simulink library "halout"  (R2021b)
settings: Solver=VariableStepAuto  StartTime=0.0  StopTime=10.0  RelTol=1e-3
undefined symbols (not defined in the file): C_TASK_5MS_S, FALSE, KHAL_CAN1TxReq_flg, KHAL_CAN2TxReq_flg, KHAL_CAN3FD3VCU1toNIDECTxReq_flg, KHAL_CAN3FD3VCU1TxReq_flg, KHAL_CAN3FD3VCU2E2E_flg, KHAL_CAN3FD3VCU2toNIDECE2E_flg, KHAL_CAN3FD3VCU2toNIDECTxReq_flg, KHAL_CAN3FD3VCU2TxReq_flg, KHAL_CAN3TxReq_flg, KHAL_CAN4FD4CE1000E2E_flg, KHAL_CAN4FD4CE1000TxReq_flg, KHAL_CAN4TxReq_flg, KHAL_CAN5TxReq_flg, KHAL_CAN7TxReq_flg, ONE_INT, TRUE, ZERO_INT
libraries: FVT_lib x258, simulink x115
(part 7 of 17)

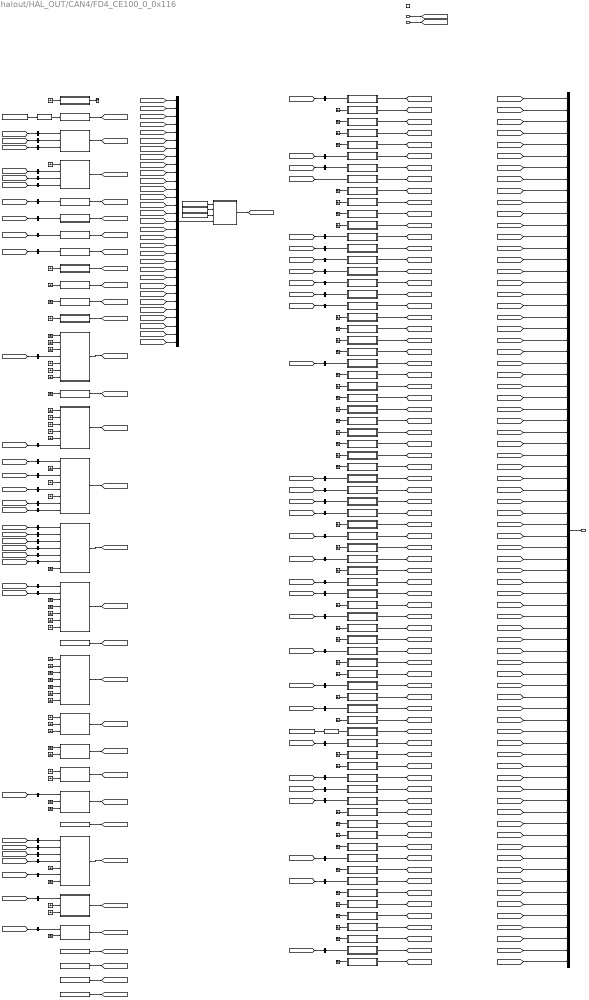
== system halout/HAL_OUT/CAN4/FD4_CE100_0_0x116 ==
  BSCP_outputs : Inport  OutDataTypeStr=Bus: BSCP_outputs
  BOUTP_outputs : Inport  Port=2  OutDataTypeStr=Bus: BOUTP_outputs
  Trigger : TriggerPort  TriggerType=function-call  VariantControl=(inherit)
  APSStaSystem : Subsystem
  AllDoorSW : Subsystem
  AntiTheftSeatFold : Subsystem
  AntitheftSta : Subsystem
  BCMDoorLockSta : Subsystem
  BrakeLamp : Subsystem
  Byte_0 : Subsystem
  Byte_1 : Subsystem
  Byte_10 : Subsystem
  Byte_11 : Subsystem
  Byte_12 : Subsystem
  Byte_13 : Subsystem
  Byte_14 : Subsystem
  Byte_15 : Subsystem
  Byte_16 : Subsystem
  Byte_17 : Subsystem
  Byte_{18,24,28..31} (6 alike) : Constant  Value=ZERO_INT
  Byte_19 : Subsystem
  Byte_2 : Subsystem
  Byte_20 : Subsystem
  Byte_21 : Subsystem
  Byte_22 : Subsystem
  Byte_23 : Subsystem
  Byte_25 : Subsystem
  Byte_26 : Subsystem
  Byte_27 : Subsystem
  Byte_3 : Subsystem
  Byte_4 : Subsystem
  Byte_5 : Subsystem
  Byte_6 : Subsystem
  Byte_7 : Subsystem
  Byte_8 : Subsystem
  Byte_9 : Subsystem
  CCCrlSta : Subsystem
  CRC8_IfAction_Tx : Subsystem  AncestorBlock=FVT_lib/hal/CRC8_IfAction_Tx
      mask help: MeasumentTrigerEvent
      mask Display: fprintf('CRC8_IfAction');
  CSVCU1CAN4 : Subsystem
  CTDCtrl : Subsystem
  CTDLockSW : Subsystem
  CTDUnlockSW : Subsystem
  Constant : Constant  Value=KHAL_CAN4FD4CE1000E2E_flg
  Constant1 : Constant  Value=0x08
  Constant2 : Constant  Value=0x4D
  Constant3 : Constant  Value=KHAL_CAN4FD4CE1000E2E_flg
  Constant4 : Constant  Value=KHAL_CAN4FD4CE1000E2E_flg
  CrashDetd : Subsystem
  CtrlDrPwrStbA2 : Subsystem
  CtrlFrBMSCCUCIR : Subsystem
  CtrlFrEDUINVERTER : Subsystem
  CtrlFrIRC1 : Subsystem
  CtrlFrPwrStbA1P : Subsystem
  DKCAuthSta : Subsystem
  DKCTimeSN : Subsystem
  Dimmer : Subsystem
  DimmerEN : Subsystem
  DoorLockIND : Subsystem
  DrDoorSW : Subsystem
  DrSeatSta : Subsystem
  EquivAccPedalSWSta : Subsystem
  FDDKCVehDataErr : Subsystem
  FDDKCVehDataSta : Subsystem
  FDTBOXDTCDataErr : Subsystem
  FDTBOXDTCDataSta : Subsystem
  FDTBOXVehDataErr : Subsystem
  FDTBOXVehDataSta : Subsystem
  FrChargingDoorCtrl : Subsystem
  FrFogLamp : Subsystem
  FrWiperH : Subsystem
  FrWiperL : Subsystem
  Ground{,1..91} (92 alike) : Ground
  HBeam : Subsystem
  HBeamADB : Subsystem
  HWResetSta : Subsystem
  HazardSW : Subsystem
  HoodSW : Subsystem
  HornCtrl : Subsystem
  LAPMWdwEnable : Subsystem
  LBSD : Subsystem
  LBeam : Subsystem
  LDRL : Subsystem
  LTurnLP : Subsystem
  LampPwr : Subsystem
  LockSetting : Subsystem
  MSACrlSta : Subsystem
  MirrorCtrl : Subsystem
  MirrorDefog : Subsystem
  Mux2 : Mux  Inputs=31
  PosLamp : Subsystem
  PsDoorSW : Subsystem
  PwrSta : Subsystem
  RBSD : Subsystem
  RCVCU1CAN4 : Subsystem
  RDRL : Subsystem
  RLDoorSW : Subsystem
  RRDoorSW : Subsystem
  RTurnLP : Subsystem
  ReBrakeLPReq : Subsystem
  ReverseLamp : Subsystem
  RollingCounter_IfAction : FVT_lib/hal/RollingCounter_IfAction
  RollingCounter_IfAction1 : FVT_lib/hal/RollingCounter_IfAction
  RoomLampH : Subsystem
  RoomLampL : Subsystem
  RrChargingDoorCtrl : Subsystem
  RrDefog : Subsystem
  RrFogLamp : Subsystem
  RrWiper : Subsystem
  ShiftGearPosn : Subsystem
  TailgateHDSW : Subsystem
  TailgateRemote : Subsystem
  TailgateSW : Subsystem
  Terminator : Terminator
  TimeSNDKCFbk : Subsystem
  TrunkRel : Subsystem
  WasherCtrl : Subsystem
  WiperFixMode : Subsystem
  bus_creator : BusCreator  Inputs=76  OutDataTypeStr=Bus: DT_CAN4_SG_FD4_CE100_0  NonVirtualBus=on
  bus_selector : BusSelector  OutputSignals=VOUTP_CCCtrlSta_enum
  bus_selector1 : BusSelector  OutputSignals=VOUTP_DrSeatSta_enum
  bus_selector10 : BusSelector  OutputSignals=VOUTP_HornCtrl_flg
  bus_selector11 : BusSelector  OutputSignals=VOUTP_RTurnLP_flg
  bus_selector12 : BusSelector  OutputSignals=VOUTP_BrakeLamp_flg
  bus_selector13 : BusSelector  OutputSignals=VOUTP_HazardSW_flg
  bus_selector14 : BusSelector  OutputSignals=VOUTP_LTurnLP_flg
  bus_selector15 : BusSelector  OutputSignals=VOUTP_ReverseLamp_flg
  bus_selector16 : BusSelector  OutputSignals=VOUTP_RrFogLamp_flg
  bus_selector17 : BusSelector  OutputSignals=VOUTP_HBeam_flg
  bus_selector18 : BusSelector  OutputSignals=VOUTP_LDRL_flg
  bus_selector19 : BusSelector  OutputSignals=VOUTP_LBeam_flg
  bus_selector2 : BusSelector  OutputSignals=VOUTP_MSACtrlSta_enum
  bus_selector20 : BusSelector  OutputSignals=VOUTP_PosLamp_flg
  bus_selector21 : BusSelector  OutputSignals=VOUTP_RDRL_flg
  bus_selector22 : BusSelector  OutputSignals=VOUTP_WasherCtrl_enum
  bus_selector23 : BusSelector  OutputSignals=VOUTP_FrWiperH_flg
  bus_selector24 : BusSelector  OutputSignals=VOUTP_FrWiperL_flg
  bus_selector25 : BusSelector  OutputSignals=VOUTP_DKCAuthSta_enum
  bus_selector26 : BusSelector  OutputSignals=VOUTP_CtrlFrBMSCCUCIR_flg
  bus_selector27 : BusSelector  OutputSignals=VOUTP_CtrlFrEDUINVERTER_flg
  bus_selector28 : BusSelector  OutputSignals=VOUTP_CtrlFrRC1_flg
  bus_selector29 : BusSelector  OutputSignals=VOUTP_CtrlFrPwrStbA1P_flg
  bus_selector3 : BusSelector  OutputSignals=VOUTP_PowerSta_enum
  bus_selector30 : BusSelector  OutputSignals=VOUTP_HWResetSta_enum
  bus_selector31 : BusSelector  OutputSignals=VOUTP_APSStaSys_enum
  bus_selector32 : BusSelector  OutputSignals=VOUTP_CtrlDrPwrStbA2_flg
  bus_selector33 : BusSelector  OutputSignals=VOUTP_APSStaSys_enum
  bus_selector34 : BusSelector  OutputSignals=VOUTP_BrakeLamp_flg
  bus_selector35 : BusSelector  OutputSignals=VOUTP_CCCtrlSta_enum
  bus_selector36 : BusSelector  OutputSignals=VOUTP_CtrlDrPwrStbA2_flg
  bus_selector37 : BusSelector  OutputSignals=VOUTP_CtrlFrBMSCCUCIR_flg
  bus_selector38 : BusSelector  OutputSignals=VOUTP_CtrlFrEDUINVERTER_flg
  bus_selector39 : BusSelector  OutputSignals=VOUTP_CtrlFrRC1_flg
  bus_selector4 : BusSelector  OutputSignals=VOUTP_ReBrakeLPReq_flg
  bus_selector40 : BusSelector  OutputSignals=VOUTP_CtrlFrPwrStbA1P_flg
  bus_selector41 : BusSelector  OutputSignals=VOUTP_DKCAuthSta_enum
  bus_selector{6..9,42} (5 alike) : BusSelector  OutputSignals=VOUTP_DKCTimeSN_cnt
  bus_selector43 : BusSelector  OutputSignals=VOUTP_DrSeatSta_enum
  bus_selector44 : BusSelector  OutputSignals=VOUTP_FrWiperH_flg
  bus_selector45 : BusSelector  OutputSignals=VOUTP_FrWiperL_flg
  bus_selector46 : BusSelector  OutputSignals=VOUTP_HWResetSta_enum
  bus_selector47 : BusSelector  OutputSignals=VOUTP_HBeam_flg
  bus_selector48 : BusSelector  OutputSignals=VOUTP_HazardSW_flg
  bus_selector49 : BusSelector  OutputSignals=VOUTP_HornCtrl_flg
  bus_selector5 : BusSelector  OutputSignals=VOUTP_ShiftGearPosn_enum
  bus_selector50 : BusSelector  OutputSignals=VOUTP_LDRL_flg
  bus_selector51 : BusSelector  OutputSignals=VOUTP_LTurnLP_flg
  bus_selector52 : BusSelector  OutputSignals=VOUTP_LBeam_flg
  bus_selector53 : BusSelector  OutputSignals=VOUTP_MSACtrlSta_enum
  bus_selector54 : BusSelector  OutputSignals=VOUTP_PosLamp_flg
  bus_selector55 : BusSelector  OutputSignals=VOUTP_PowerSta_enum
  bus_selector56 : BusSelector  OutputSignals=VOUTP_RDRL_flg
  bus_selector57 : BusSelector  OutputSignals=VOUTP_RTurnLP_flg
  bus_selector58 : BusSelector  OutputSignals=VOUTP_ReBrakeLPReq_flg
  bus_selector59 : BusSelector  OutputSignals=VOUTP_ReverseLamp_flg
  bus_selector60 : BusSelector  OutputSignals=VOUTP_RrFogLamp_flg
  bus_selector61 : BusSelector  OutputSignals=VOUTP_ShiftGearPosn_enum
  bus_selector62 : BusSelector  OutputSignals=VOUTP_WasherCtrl_enum
  FD4_CE100_0 : Outport
  wires:
  BSCP_outputs/1 -> [BSCP_outputs]
  BOUTP_outputs/1 -> [BOUTP_outputs]
  [CAN4_APS_Sta_System] -> bus_creator/1  "CAN4_APS_Sta_System"
  [CAN4_AllDoorSW] -> bus_creator/2  "CAN4_AllDoorSW"
  [CAN4_AntiTheftSeatFold] -> bus_creator/3  "CAN4_AntiTheftSeatFold"
  [CAN4_AntitheftSta] -> bus_creator/4  "CAN4_AntitheftSta"
  [CAN4_BCM_DoorLock_Sta] -> bus_creator/5  "CAN4_BCM_DoorLock_Sta"
  [CAN4_BrakeLamp] -> bus_creator/6  "CAN4_BrakeLamp"
  [CAN4_CC_Crl_Sta] -> bus_creator/7  "CAN4_CC_Crl_Sta"
  [CAN4_CS_VCU1_CAN4] -> bus_creator/8  "CAN4_CS_VCU1_CAN4"
  [CAN4_CTDCtrl] -> bus_creator/9  "CAN4_CTDCtrl"
  [CAN4_CTDLockSW] -> bus_creator/10  "CAN4_CTDLockSW"
  [CAN4_CTDUnlockSW] -> bus_creator/11  "CAN4_CTDUnlockSW"
  [CAN4_CrashDetd] -> bus_creator/12  "CAN4_CrashDetd"
  [CAN4_CtrlDrPwrStbA2] -> bus_creator/13  "CAN4_CtrlDrPwrStbA2"
  [CAN4_CtrlFrBMSCCUCIR] -> bus_creator/14  "CAN4_CtrlFrBMSCCUCIR"
  [CAN4_CtrlFrEDUINVERTER] -> bus_creator/15  "CAN4_CtrlFrEDUINVERTER"
  [CAN4_CtrlFrIRC1] -> bus_creator/16  "CAN4_CtrlFrIRC1"
  [CAN4_CtrlFrPwrStbA1P] -> bus_creator/17  "CAN4_CtrlFrPwrStbA1P"
  [CAN4_DKCAuthSta] -> bus_creator/18  "CAN4_DKCAuthSta"
  [CAN4_DKCTimeSN] -> bus_creator/19  "CAN4_DKCTimeSN"
  [CAN4_Dimmer] -> bus_creator/20  "CAN4_Dimmer"
  [CAN4_DimmerEN] -> bus_creator/21  "CAN4_DimmerEN"
  [CAN4_DoorLockIND] -> bus_creator/22  "CAN4_DoorLockIND"
  [CAN4_DrDoorSW] -> bus_creator/23  "CAN4_DrDoorSW"
  [CAN4_Dr_SeatSta] -> bus_creator/24  "CAN4_Dr_SeatSta"
  [CAN4_EquivAccPedalSWSta] -> bus_creator/25  "CAN4_EquivAccPedalSWSta"
  [CAN4_FD_DKC_VehData_Err] -> bus_creator/26  "CAN4_FD_DKC_VehData_Err"
  [CAN4_FD_DKC_VehData_Sta] -> bus_creator/27  "CAN4_FD_DKC_VehData_Sta"
  [CAN4_FD_TBOX_DTCData_Err] -> bus_creator/28  "CAN4_FD_TBOX_DTCData_Err"
  [CAN4_FD_TBOX_DTCData_Sta] -> bus_creator/29  "CAN4_FD_TBOX_DTCData_Sta"
  [CAN4_FD_TBOX_VehData_Err] -> bus_creator/30  "CAN4_FD_TBOX_VehData_Err"
  [CAN4_FD_TBOX_VehData_Sta] -> bus_creator/31  "CAN4_FD_TBOX_VehData_Sta"
  [CAN4_Fr_ChargingDoorCtrl] -> bus_creator/32  "CAN4_Fr_ChargingDoorCtrl"
  [CAN4_Fr_FogLamp] -> bus_creator/33  "CAN4_Fr_FogLamp"
  [CAN4_Fr_Wiper_H] -> bus_creator/34  "CAN4_Fr_Wiper_H"
  [CAN4_Fr_Wiper_L] -> bus_creator/35  "CAN4_Fr_Wiper_L"
  [CAN4_HWResetSta] -> bus_creator/36  "CAN4_HWResetSta"
  [CAN4_H_Beam] -> bus_creator/37  "CAN4_H_Beam"
  [CAN4_H_Beam_ADB] -> bus_creator/38  "CAN4_H_Beam_ADB"
  [CAN4_HazardSW] -> bus_creator/39  "CAN4_HazardSW"
  [CAN4_HoodSW] -> bus_creator/40  "CAN4_HoodSW"
  [CAN4_HornCtrl] -> bus_creator/41  "CAN4_HornCtrl"
  [CAN4_LBSD] -> bus_creator/42  "CAN4_LBSD"
  [CAN4_LDRL] -> bus_creator/43  "CAN4_LDRL"
  [CAN4_LTurnLP] -> bus_creator/44  "CAN4_LTurnLP"
  [CAN4_L_APM_WdwEnable] -> bus_creator/45  "CAN4_L_APM_WdwEnable"
  [CAN4_L_Beam] -> bus_creator/46  "CAN4_L_Beam"
  [CAN4_LampPwr] -> bus_creator/47  "CAN4_LampPwr"
  [CAN4_LockSetting] -> bus_creator/48  "CAN4_LockSetting"
  [CAN4_MSA_Crl_Sta] -> bus_creator/49  "CAN4_MSA_Crl_Sta"
  [CAN4_MirrorCtrl] -> bus_creator/50  "CAN4_MirrorCtrl"
  [CAN4_MirrorDefog] -> bus_creator/51  "CAN4_MirrorDefog"
  [CAN4_PosLamp] -> bus_creator/52  "CAN4_PosLamp"
  [CAN4_PsDoorSW] -> bus_creator/53  "CAN4_PsDoorSW"
  [CAN4_PwrSta] -> bus_creator/54  "CAN4_PwrSta"
  [CAN4_RBSD] -> bus_creator/55  "CAN4_RBSD"
  [CAN4_RC_VCU1_CAN4] -> bus_creator/56  "CAN4_RC_VCU1_CAN4"
  [CAN4_RDRL] -> bus_creator/57  "CAN4_RDRL"
  [CAN4_RLDoorSW] -> bus_creator/58  "CAN4_RLDoorSW"
  [CAN4_RRDoorSW] -> bus_creator/59  "CAN4_RRDoorSW"
  [CAN4_RTurnLP] -> bus_creator/60  "CAN4_RTurnLP"
  [CAN4_ReBrakeLPReq] -> bus_creator/61  "CAN4_ReBrakeLPReq"
  [CAN4_ReverseLamp] -> bus_creator/62  "CAN4_ReverseLamp"
  [CAN4_RoomLampH] -> bus_creator/63  "CAN4_RoomLampH"
  [CAN4_RoomLampL] -> bus_creator/64  "CAN4_RoomLampL"
  [CAN4_Rr_ChargingDoorCtrl] -> bus_creator/65  "CAN4_Rr_ChargingDoorCtrl"
  [CAN4_Rr_Defog] -> bus_creator/66  "CAN4_Rr_Defog"
  [CAN4_Rr_FogLamp] -> bus_creator/67  "CAN4_Rr_FogLamp"
  [CAN4_Rr_Wiper] -> bus_creator/68  "CAN4_Rr_Wiper"
  [CAN4_ShiftGearPosn] -> bus_creator/69  "CAN4_ShiftGearPosn"
  [CAN4_TailgateHDSW] -> bus_creator/70  "CAN4_TailgateHDSW"
  [CAN4_TailgateRemote] -> bus_creator/71  "CAN4_TailgateRemote"
  [CAN4_Tailgate_SW] -> bus_creator/72  "CAN4_Tailgate_SW"
  [CAN4_TimeSNDKCFbk] -> bus_creator/73  "CAN4_TimeSNDKCFbk"
  [CAN4_TrunkRel] -> bus_creator/74  "CAN4_TrunkRel"
  [CAN4_WasherCtrl] -> bus_creator/75  "CAN4_WasherCtrl"
  [CAN4_WiperFixMode] -> bus_creator/76  "CAN4_WiperFixMode"
  bus_creator/1 -> FD4_CE100_0/1
  APSStaSystem/1(CAN4_APS_Sta_System) -> [CAN4_APS_Sta_System]
  AllDoorSW/1(CAN4_AllDoorSW) -> [CAN4_AllDoorSW]
  AntiTheftSeatFold/1(CAN4_AntiTheftSeatFold) -> [CAN4_AntiTheftSeatFold]
  AntitheftSta/1(CAN4_AntitheftSta) -> [CAN4_AntitheftSta]
  BCMDoorLockSta/1(CAN4_BCM_DoorLock_Sta) -> [CAN4_BCM_DoorLock_Sta]
  BrakeLamp/1(CAN4_BrakeLamp) -> [CAN4_BrakeLamp]
  CCCrlSta/1(CAN4_CC_Crl_Sta) -> [CAN4_CC_Crl_Sta]
  CSVCU1CAN4/1(CAN4_CS_VCU1_CAN4) -> [CAN4_CS_VCU1_CAN4]
  CTDCtrl/1(CAN4_CTDCtrl) -> [CAN4_CTDCtrl]
  CTDLockSW/1(CAN4_CTDLockSW) -> [CAN4_CTDLockSW]
  CTDUnlockSW/1(CAN4_CTDUnlockSW) -> [CAN4_CTDUnlockSW]
  CrashDetd/1(CAN4_CrashDetd) -> [CAN4_CrashDetd]
  CtrlDrPwrStbA2/1(CAN4_CtrlDrPwrStbA2) -> [CAN4_CtrlDrPwrStbA2]
  CtrlFrBMSCCUCIR/1(CAN4_CtrlFrBMSCCUCIR) -> [CAN4_CtrlFrBMSCCUCIR]
  CtrlFrEDUINVERTER/1(CAN4_CtrlFrEDUINVERTER) -> [CAN4_CtrlFrEDUINVERTER]
  CtrlFrIRC1/1(CAN4_CtrlFrIRC1) -> [CAN4_CtrlFrIRC1]
  CtrlFrPwrStbA1P/1(CAN4_CtrlFrPwrStbA1P) -> [CAN4_CtrlFrPwrStbA1P]
  DKCAuthSta/1(CAN4_DKCAuthSta) -> [CAN4_DKCAuthSta]
  DKCTimeSN/1(CAN4_DKCTimeSN) -> [CAN4_DKCTimeSN]
  Dimmer/1(CAN4_Dimmer) -> [CAN4_Dimmer]
  DimmerEN/1(CAN4_DimmerEN) -> [CAN4_DimmerEN]
  DoorLockIND/1(CAN4_DoorLockIND) -> [CAN4_DoorLockIND]
  DrDoorSW/1(CAN4_DrDoorSW) -> [CAN4_DrDoorSW]
  DrSeatSta/1(CAN4_Dr_SeatSta) -> [CAN4_Dr_SeatSta]
  EquivAccPedalSWSta/1(CAN4_EquivAccPedalSWSta) -> [CAN4_EquivAccPedalSWSta]
  FDDKCVehDataErr/1(CAN4_FD_DKC_VehData_Err) -> [CAN4_FD_DKC_VehData_Err]
  FDDKCVehDataSta/1(CAN4_FD_DKC_VehData_Sta) -> [CAN4_FD_DKC_VehData_Sta]
  FDTBOXDTCDataErr/1(CAN4_FD_TBOX_DTCData_Err) -> [CAN4_FD_TBOX_DTCData_Err]
  FDTBOXDTCDataSta/1(CAN4_FD_TBOX_DTCData_Sta) -> [CAN4_FD_TBOX_DTCData_Sta]
  FDTBOXVehDataErr/1(CAN4_FD_TBOX_VehData_Err) -> [CAN4_FD_TBOX_VehData_Err]
  FDTBOXVehDataSta/1(CAN4_FD_TBOX_VehData_Sta) -> [CAN4_FD_TBOX_VehData_Sta]
  FrChargingDoorCtrl/1(CAN4_Fr_ChargingDoorCtrl) -> [CAN4_Fr_ChargingDoorCtrl]
  FrFogLamp/1(CAN4_Fr_FogLamp) -> [CAN4_Fr_FogLamp]
  FrWiperH/1(CAN4_Fr_Wiper_H) -> [CAN4_Fr_Wiper_H]
  FrWiperL/1(CAN4_Fr_Wiper_L) -> [CAN4_Fr_Wiper_L]
  HWResetSta/1(CAN4_HWResetSta) -> [CAN4_HWResetSta]
  HBeam/1(CAN4_H_Beam) -> [CAN4_H_Beam]
  HBeamADB/1(CAN4_H_Beam_ADB) -> [CAN4_H_Beam_ADB]
  HazardSW/1(CAN4_HazardSW) -> [CAN4_HazardSW]
  HoodSW/1(CAN4_HoodSW) -> [CAN4_HoodSW]
  HornCtrl/1(CAN4_HornCtrl) -> [CAN4_HornCtrl]
  LBSD/1(CAN4_LBSD) -> [CAN4_LBSD]
  LDRL/1(CAN4_LDRL) -> [CAN4_LDRL]
  LTurnLP/1(CAN4_LTurnLP) -> [CAN4_LTurnLP]
  LAPMWdwEnable/1(CAN4_L_APM_WdwEnable) -> [CAN4_L_APM_WdwEnable]
  LBeam/1(CAN4_L_Beam) -> [CAN4_L_Beam]
  LampPwr/1(CAN4_LampPwr) -> [CAN4_LampPwr]
  LockSetting/1(CAN4_LockSetting) -> [CAN4_LockSetting]
  MSACrlSta/1(CAN4_MSA_Crl_Sta) -> [CAN4_MSA_Crl_Sta]
  MirrorCtrl/1(CAN4_MirrorCtrl) -> [CAN4_MirrorCtrl]
  MirrorDefog/1(CAN4_MirrorDefog) -> [CAN4_MirrorDefog]
  PosLamp/1(CAN4_PosLamp) -> [CAN4_PosLamp]
  PsDoorSW/1(CAN4_PsDoorSW) -> [CAN4_PsDoorSW]
  PwrSta/1(CAN4_PwrSta) -> [CAN4_PwrSta]
  RBSD/1(CAN4_RBSD) -> [CAN4_RBSD]
  RCVCU1CAN4/1(CAN4_RC_VCU1_CAN4) -> [CAN4_RC_VCU1_CAN4]
  RDRL/1(CAN4_RDRL) -> [CAN4_RDRL]
  RLDoorSW/1(CAN4_RLDoorSW) -> [CAN4_RLDoorSW]
  RRDoorSW/1(CAN4_RRDoorSW) -> [CAN4_RRDoorSW]
  RTurnLP/1(CAN4_RTurnLP) -> [CAN4_RTurnLP]
  ReBrakeLPReq/1(CAN4_ReBrakeLPReq) -> [CAN4_ReBrakeLPReq]
  ReverseLamp/1(CAN4_ReverseLamp) -> [CAN4_ReverseLamp]
  RoomLampH/1(CAN4_RoomLampH) -> [CAN4_RoomLampH]
  RoomLampL/1(CAN4_RoomLampL) -> [CAN4_RoomLampL]
  RrChargingDoorCtrl/1(CAN4_Rr_ChargingDoorCtrl) -> [CAN4_Rr_ChargingDoorCtrl]
  RrDefog/1(CAN4_Rr_Defog) -> [CAN4_Rr_Defog]
  RrFogLamp/1(CAN4_Rr_FogLamp) -> [CAN4_Rr_FogLamp]
  RrWiper/1(CAN4_Rr_Wiper) -> [CAN4_Rr_Wiper]
  ShiftGearPosn/1(CAN4_ShiftGearPosn) -> [CAN4_ShiftGearPosn]
  TailgateHDSW/1(CAN4_TailgateHDSW) -> [CAN4_TailgateHDSW]
  TailgateRemote/1(CAN4_TailgateRemote) -> [CAN4_TailgateRemote]
  TailgateSW/1(CAN4_Tailgate_SW) -> [CAN4_Tailgate_SW]
  TimeSNDKCFbk/1(CAN4_TimeSNDKCFbk) -> [CAN4_TimeSNDKCFbk]
  TrunkRel/1(CAN4_TrunkRel) -> [CAN4_TrunkRel]
  WasherCtrl/1(CAN4_WasherCtrl) -> [CAN4_WasherCtrl]
  WiperFixMode/1(CAN4_WiperFixMode) -> [CAN4_WiperFixMode]
  Byte_0/1(Byte_0) -> Terminator/1
  Byte_1/1(Byte_1) -> [Byte_1]
  Byte_2/1(Byte_2) -> [Byte_2]
  Byte_3/1(Byte_3) -> [Byte_3]
  Byte_4/1(Byte_4) -> [Byte_4]
  Byte_5/1(Byte_5) -> [Byte_5]
  Byte_6/1(Byte_6) -> [Byte_6]
  Byte_7/1(Byte_7) -> [Byte_7]
  Byte_8/1(Byte_8) -> [Byte_8]
  Byte_9/1(Byte_9) -> [Byte_9]
  Byte_10/1(Byte_10) -> [Byte_10]
  Byte_11/1(Byte_11) -> [Byte_11]
  Byte_12/1(Byte_12) -> [Byte_12]
  Byte_13/1(Byte_13) -> [Byte_13]
  Byte_14/1(Byte_14) -> [Byte_14]
  Byte_15/1(Byte_15) -> [Byte_15]
  Byte_16/1(Byte_16) -> [Byte_16]
  Byte_17/1(Byte_17) -> [Byte_17]
  Byte_18/1 -> [Byte_18]
  Byte_19/1(Byte_19) -> [Byte_19]
  Byte_20/1(Byte_20) -> [Byte_20]
  Byte_21/1(Byte_21) -> [Byte_21]
  Byte_22/1(Byte_22) -> [Byte_22]
  Byte_23/1(Byte_23) -> [Byte_23]
  Byte_24/1 -> [Byte_24]
  Byte_25/1(Byte_25) -> [Byte_25]
  Byte_26/1(Byte_26) -> [Byte_26]
  Byte_27/1(Byte_27) -> [Byte_27]
  Byte_28/1 -> [Byte_28]
  Byte_29/1 -> [Byte_29]
  Byte_30/1 -> [Byte_30]
  Byte_31/1 -> [Byte_31]
  Mux2/1 -> CRC8_IfAction_Tx/4(RawData)
  Constant/1 -> CRC8_IfAction_Tx/1(CAN_E2E_flg)
  Constant1/1 -> CRC8_IfAction_Tx/2(DataID1)
  Constant2/1 -> CRC8_IfAction_Tx/3(DataID2)
  CRC8_IfAction_Tx/1(CRC8) -> [CS_VCU1_CAN4]
  Ground/1 -> Byte_0/1(CS_VCU1_CAN4)
  [Byte_1] -> Mux2/1
  RollingCounter_IfAction/1 -> Byte_1/1(RC_VCU1_CAN4)
  Constant3/1 -> RollingCounter_IfAction/1
  [Byte_2] -> Mux2/2
  bus_selector/1 -> Byte_2/1(CC_Crl_Sta)  "<VOUTP_CCCtrlSta_enum>"
  [BOUTP_outputs] -> bus_selector/1
  bus_selector1/1 -> Byte_2/2(Dr_SeatSta)  "<VOUTP_DrSeatSta_enum>"
  [BOUTP_outputs] -> bus_selector1/1
  bus_selector2/1 -> Byte_2/3(MSA_Crl_Sta)  "<VOUTP_MSACtrlSta_enum>"
  [BOUTP_outputs] -> bus_selector2/1
  [Byte_3] -> Mux2/3
  Ground1/1 -> Byte_3/1(H_Beam_ADB)
  bus_selector3/1 -> Byte_3/2(PwrSta)  "<VOUTP_PowerSta_enum>"
  [BOUTP_outputs] -> bus_selector3/1
  bus_selector4/1 -> Byte_3/3(ReBrakeLPReq)  "<VOUTP_ReBrakeLPReq_flg>"
  [BOUTP_outputs] -> bus_selector4/1
  bus_selector5/1 -> Byte_3/4(ShiftGearPosn)  "<VOUTP_ShiftGearPosn_enum>"
  [BOUTP_outputs] -> bus_selector5/1
  [Byte_4] -> Mux2/4
  bus_selector6/1 -> Byte_4/1(DKCTimeSN)  "<VOUTP_DKCTimeSN_cnt>"
  [BOUTP_outputs] -> bus_selector6/1
  [Byte_5] -> Mux2/5
  bus_selector7/1 -> Byte_5/1(DKCTimeSN)  "<VOUTP_DKCTimeSN_cnt>"
  [BOUTP_outputs] -> bus_selector7/1
  [Byte_6] -> Mux2/6
  bus_selector8/1 -> Byte_6/1(DKCTimeSN)  "<VOUTP_DKCTimeSN_cnt>"
  [BOUTP_outputs] -> bus_selector8/1
  [Byte_7] -> Mux2/7
  bus_selector9/1 -> Byte_7/1(DKCTimeSN)  "<VOUTP_DKCTimeSN_cnt>"
  [BOUTP_outputs] -> bus_selector9/1
  [Byte_8] -> Mux2/8
  Ground2/1 -> Byte_8/1(TimeSNDKCFbk)
  [Byte_9] -> Mux2/9
  Ground3/1 -> Byte_9/1(TimeSNDKCFbk)
  [Byte_10] -> Mux2/10
  Ground4/1 -> Byte_10/1(TimeSNDKCFbk)
  [Byte_11] -> Mux2/11
  Ground5/1 -> Byte_11/1(TimeSNDKCFbk)
  [Byte_12] -> Mux2/12
  Ground6/1 -> Byte_12/1(BCM_DoorLock_Sta)
  Ground7/1 -> Byte_12/2(DimmerEN)
  Ground8/1 -> Byte_12/3(EquivAccPedalSWSta)
  bus_selector10/1 -> Byte_12/4(HornCtrl)  "<VOUTP_HornCtrl_flg>"
  [BOUTP_outputs] -> bus_selector10/1
  Ground9/1 -> Byte_12/5(RoomLampH)
  Ground10/1 -> Byte_12/6(RoomLampL)
  Ground11/1 -> Byte_12/7(TailgateRemote)
  [Byte_13] -> Mux2/13
  Ground12/1 -> Byte_13/1(Dimmer)
  [Byte_14] -> Mux2/14
  Ground13/1 -> Byte_14/1(AntiTheftSeatFold)
  Ground14/1 -> Byte_14/2(AntitheftSta)
  Ground15/1 -> Byte_14/3(CrashDetd)
  Ground16/1 -> Byte_14/4(L_APM_WdwEnable)
  Ground17/1 -> Byte_14/5(LockSetting)
  bus_selector11/1 -> Byte_14/6(RTurnLP)  "<VOUTP_RTurnLP_flg>"
  [BOUTP_outputs] -> bus_selector11/1
  [Byte_15] -> Mux2/15
  bus_selector12/1 -> Byte_15/1(BrakeLamp)  "<VOUTP_BrakeLamp_flg>"
  [BOUTP_outputs] -> bus_selector12/1
  Ground18/1 -> Byte_15/2(Fr_FogLamp)
  bus_selector13/1 -> Byte_15/3(HazardSW)  "<VOUTP_HazardSW_flg>"
  [BOUTP_outputs] -> bus_selector13/1
  Ground19/1 -> Byte_15/4(LBSD)
  bus_selector14/1 -> Byte_15/5(LTurnLP)  "<VOUTP_LTurnLP_flg>"
  [BOUTP_outputs] -> bus_selector14/1
  Ground20/1 -> Byte_15/6(RBSD)
  bus_selector15/1 -> Byte_15/7(ReverseLamp)  "<VOUTP_ReverseLamp_flg>"
  [BOUTP_outputs] -> bus_selector15/1
  bus_selector16/1 -> Byte_15/8(Rr_FogLamp)  "<VOUTP_RrFogLamp_flg>"
  [BOUTP_outputs] -> bus_selector16/1
  [Byte_16] -> Mux2/16
  bus_selector17/1 -> Byte_16/1(H_Beam)  "<VOUTP_HBeam_flg>"
  [BOUTP_outputs] -> bus_selector17/1
  bus_selector18/1 -> Byte_16/2(LDRL)  "<VOUTP_LDRL_flg>"
  [BOUTP_outputs] -> bus_selector18/1
  bus_selector19/1 -> Byte_16/3(L_Beam)  "<VOUTP_LBeam_flg>"
  [BOUTP_outputs] -> bus_selector19/1
  bus_selector20/1 -> Byte_16/4(PosLamp)  "<VOUTP_PosLamp_flg>"
  [BOUTP_outputs] -> bus_selector20/1
  bus_selector21/1 -> Byte_16/5(RDRL)  "<VOUTP_RDRL_flg>"
  [BOUTP_outputs] -> bus_selector21/1
  bus_selector22/1 -> Byte_16/6(WasherCtrl)  "<VOUTP_WasherCtrl_enum>"
  [BOUTP_outputs] -> bus_selector22/1
  Ground21/1 -> Byte_16/7(WiperFixMode)
  [Byte_17] -> Mux2/17
  bus_selector23/1 -> Byte_17/1(Fr_Wiper_H)  "<VOUTP_FrWiperH_flg>"
  [BOUTP_outputs] -> bus_selector23/1
  bus_selector24/1 -> Byte_17/2(Fr_Wiper_L)  "<VOUTP_FrWiperL_flg>"
  [BOUTP_outputs] -> bus_selector24/1
  Ground22/1 -> Byte_17/3(MirrorCtrl)
  Ground23/1 -> Byte_17/4(Rr_Defog)
  Ground24/1 -> Byte_17/5(Rr_Wiper)
  Ground25/1 -> Byte_17/6(TailgateHDSW)
  Ground26/1 -> Byte_17/7(TrunkRel)
  [Byte_18] -> Mux2/18
  [Byte_19] -> Mux2/19
  Ground27/1 -> Byte_19/1(AllDoorSW)
  Ground28/1 -> Byte_19/2(DoorLockIND)
  Ground29/1 -> Byte_19/3(Fr_ChargingDoorCtrl)
  Ground30/1 -> Byte_19/4(HoodSW)
  Ground31/1 -> Byte_19/5(PsDoorSW)
  Ground32/1 -> Byte_19/6(RLDoorSW)
  Ground33/1 -> Byte_19/7(RRDoorSW)
  [Byte_20] -> Mux2/20
  Ground34/1 -> Byte_20/1(CTDCtrl)
  Ground35/1 -> Byte_20/2(FD_TBOX_VehData_Sta)
  Ground36/1 -> Byte_20/3(Rr_ChargingDoorCtrl)
  [Byte_21] -> Mux2/21
  Ground37/1 -> Byte_21/1(FD_DKC_VehData_Sta)
  Ground38/1 -> Byte_21/2(FD_TBOX_VehData_Err)
  [Byte_22] -> Mux2/22
  Ground39/1 -> Byte_22/1(FD_DKC_VehData_Err)
  Ground40/1 -> Byte_22/2(FD_TBOX_DTCData_Sta)
  [Byte_23] -> Mux2/23
  bus_selector25/1 -> Byte_23/1(DKCAuthSta)  "<VOUTP_DKCAuthSta_enum>"
  [BOUTP_outputs] -> bus_selector25/1
  Ground41/1 -> Byte_23/2(FD_TBOX_DTCData_Err)
  Ground42/1 -> Byte_23/3(LampPwr)
  [Byte_24] -> Mux2/24
  [Byte_25] -> Mux2/25
  bus_selector26/1 -> Byte_25/1(CtrlFrBMSCCUCIR)  "<VOUTP_CtrlFrBMSCCUCIR_flg>"
  [BOUTP_outputs] -> bus_selector26/1
  bus_selector27/1 -> Byte_25/2(CtrlFrEDUINVERTER)  "<VOUTP_CtrlFrEDUINVERTER_flg>"
  [BOUTP_outputs] -> bus_selector27/1
  bus_selector28/1 -> Byte_25/3(CtrlFrIRC1)  "<VOUTP_CtrlFrRC1_flg>"
  [BOUTP_outputs] -> bus_selector28/1
  bus_selector29/1 -> Byte_25/4(CtrlFrPwrStbA1P)  "<VOUTP_CtrlFrPwrStbA1P_flg>"
  [BOUTP_outputs] -> bus_selector29/1
  Ground43/1 -> Byte_25/5(DrDoorSW)
  bus_selector30/1 -> Byte_25/6(HWResetSta)  "<VOUTP_HWResetSta_enum>"
  [BOUTP_outputs] -> bus_selector30/1
  Ground44/1 -> Byte_25/7(MirrorDefog)
  [Byte_26] -> Mux2/26
  bus_selector31/1 -> Byte_26/1(APS_Sta_System)  "<VOUTP_APSStaSys_enum>"
  [BOUTP_outputs] -> bus_selector31/1
  Ground45/1 -> Byte_26/2(CTDLockSW)
  Ground46/1 -> Byte_26/3(CTDUnlockSW)
  [Byte_27] -> Mux2/27
  bus_selector32/1 -> Byte_27/1(CtrlDrPwrStbA2)  "<VOUTP_CtrlDrPwrStbA2_flg>"
  [BOUTP_outputs] -> bus_selector32/1
  Ground47/1 -> Byte_27/2(Tailgate_SW)
  [Byte_28] -> Mux2/28
  [Byte_29] -> Mux2/29
  [Byte_30] -> Mux2/30
  [Byte_31] -> Mux2/31
  bus_selector33/1 -> APSStaSystem/1(APSStaSystem)  "<VOUTP_APSStaSys_enum>"
  [BOUTP_outputs] -> bus_selector33/1
  Ground48/1 -> AllDoorSW/1(AllDoorSW)
  Ground49/1 -> AntiTheftSeatFold/1(AntiTheftSeatFold)
  Ground50/1 -> AntitheftSta/1(AntitheftSta)
  Ground51/1 -> BCMDoorLockSta/1(BCMDoorLockSta)
  bus_selector34/1 -> BrakeLamp/1(BrakeLamp)  "<VOUTP_BrakeLamp_flg>"
  [BOUTP_outputs] -> bus_selector34/1
  bus_selector35/1 -> CCCrlSta/1(CCCrlSta)  "<VOUTP_CCCtrlSta_enum>"
  [BOUTP_outputs] -> bus_selector35/1
  [CS_VCU1_CAN4] -> CSVCU1CAN4/1(CSVCU1CAN4)
  Ground52/1 -> CTDCtrl/1(CTDCtrl)
  Ground53/1 -> CTDLockSW/1(CTDLockSW)
  Ground54/1 -> CTDUnlockSW/1(CTDUnlockSW)
  Ground55/1 -> CrashDetd/1(CrashDetd)
  bus_selector36/1 -> CtrlDrPwrStbA2/1(CtrlDrPwrStbA2)  "<VOUTP_CtrlDrPwrStbA2_flg>"
  [BOUTP_outputs] -> bus_selector36/1
  bus_selector37/1 -> CtrlFrBMSCCUCIR/1(CtrlFrBMSCCUCIR)  "<VOUTP_CtrlFrBMSCCUCIR_flg>"
  [BOUTP_outputs] -> bus_selector37/1
  bus_selector38/1 -> CtrlFrEDUINVERTER/1(CtrlFrEDUINVERTER)  "<VOUTP_CtrlFrEDUINVERTER_flg>"
  [BOUTP_outputs] -> bus_selector38/1
  bus_selector39/1 -> CtrlFrIRC1/1(CtrlFrIRC1)  "<VOUTP_CtrlFrRC1_flg>"
  [BOUTP_outputs] -> bus_selector39/1
  bus_selector40/1 -> CtrlFrPwrStbA1P/1(CtrlFrPwrStbA1P)  "<VOUTP_CtrlFrPwrStbA1P_flg>"
  [BOUTP_outputs] -> bus_selector40/1
  bus_selector41/1 -> DKCAuthSta/1(DKCAuthSta)  "<VOUTP_DKCAuthSta_enum>"
  [BOUTP_outputs] -> bus_selector41/1
  bus_selector42/1 -> DKCTimeSN/1(DKCTimeSN)  "<VOUTP_DKCTimeSN_cnt>"
  [BOUTP_outputs] -> bus_selector42/1
  Ground56/1 -> Dimmer/1(Dimmer)
  Ground57/1 -> DimmerEN/1(DimmerEN)
  Ground58/1 -> DoorLockIND/1(DoorLockIND)
  Ground59/1 -> DrDoorSW/1(DrDoorSW)
  bus_selector43/1 -> DrSeatSta/1(DrSeatSta)  "<VOUTP_DrSeatSta_enum>"
  [BOUTP_outputs] -> bus_selector43/1
  Ground60/1 -> EquivAccPedalSWSta/1(EquivAccPedalSWSta)
  Ground61/1 -> FDDKCVehDataErr/1(FDDKCVehDataErr)
  Ground62/1 -> FDDKCVehDataSta/1(FDDKCVehDataSta)
  Ground63/1 -> FDTBOXDTCDataErr/1(FDTBOXDTCDataErr)
  Ground64/1 -> FDTBOXDTCDataSta/1(FDTBOXDTCDataSta)
  Ground65/1 -> FDTBOXVehDataErr/1(FDTBOXVehDataErr)
  Ground66/1 -> FDTBOXVehDataSta/1(FDTBOXVehDataSta)
  Ground67/1 -> FrChargingDoorCtrl/1(FrChargingDoorCtrl)
  Ground68/1 -> FrFogLamp/1(FrFogLamp)
  bus_selector44/1 -> FrWiperH/1(FrWiperH)  "<VOUTP_FrWiperH_flg>"
  [BOUTP_outputs] -> bus_selector44/1
  bus_selector45/1 -> FrWiperL/1(FrWiperL)  "<VOUTP_FrWiperL_flg>"
  [BOUTP_outputs] -> bus_selector45/1
  bus_selector46/1 -> HWResetSta/1(HWResetSta)  "<VOUTP_HWResetSta_enum>"
  [BOUTP_outputs] -> bus_selector46/1
  bus_selector47/1 -> HBeam/1(HBeam)  "<VOUTP_HBeam_flg>"
  [BOUTP_outputs] -> bus_selector47/1
  Ground69/1 -> HBeamADB/1(HBeamADB)
  bus_selector48/1 -> HazardSW/1(HazardSW)  "<VOUTP_HazardSW_flg>"
  [BOUTP_outputs] -> bus_selector48/1
  Ground70/1 -> HoodSW/1(HoodSW)
  bus_selector49/1 -> HornCtrl/1(HornCtrl)  "<VOUTP_HornCtrl_flg>"
  [BOUTP_outputs] -> bus_selector49/1
  Ground71/1 -> LBSD/1(LBSD)
  bus_selector50/1 -> LDRL/1(LDRL)  "<VOUTP_LDRL_flg>"
  [BOUTP_outputs] -> bus_selector50/1
  bus_selector51/1 -> LTurnLP/1(LTurnLP)  "<VOUTP_LTurnLP_flg>"
  [BOUTP_outputs] -> bus_selector51/1
  Ground72/1 -> LAPMWdwEnable/1(LAPMWdwEnable)
  bus_selector52/1 -> LBeam/1(LBeam)  "<VOUTP_LBeam_flg>"
  [BOUTP_outputs] -> bus_selector52/1
  Ground73/1 -> LampPwr/1(LampPwr)
  Ground74/1 -> LockSetting/1(LockSetting)
  bus_selector53/1 -> MSACrlSta/1(MSACrlSta)  "<VOUTP_MSACtrlSta_enum>"
  [BOUTP_outputs] -> bus_selector53/1
  Ground75/1 -> MirrorCtrl/1(MirrorCtrl)
  Ground76/1 -> MirrorDefog/1(MirrorDefog)
  bus_selector54/1 -> PosLamp/1(PosLamp)  "<VOUTP_PosLamp_flg>"
  [BOUTP_outputs] -> bus_selector54/1
  Ground77/1 -> PsDoorSW/1(PsDoorSW)
  bus_selector55/1 -> PwrSta/1(PwrSta)  "<VOUTP_PowerSta_enum>"
  [BOUTP_outputs] -> bus_selector55/1
  Ground78/1 -> RBSD/1(RBSD)
  RollingCounter_IfAction1/1 -> RCVCU1CAN4/1(RCVCU1CAN4)
  Constant4/1 -> RollingCounter_IfAction1/1
  bus_selector56/1 -> RDRL/1(RDRL)  "<VOUTP_RDRL_flg>"
  [BOUTP_outputs] -> bus_selector56/1
  Ground79/1 -> RLDoorSW/1(RLDoorSW)
  Ground80/1 -> RRDoorSW/1(RRDoorSW)
  bus_selector57/1 -> RTurnLP/1(RTurnLP)  "<VOUTP_RTurnLP_flg>"
  [BOUTP_outputs] -> bus_selector57/1
  bus_selector58/1 -> ReBrakeLPReq/1(ReBrakeLPReq)  "<VOUTP_ReBrakeLPReq_flg>"
  [BOUTP_outputs] -> bus_selector58/1
  bus_selector59/1 -> ReverseLamp/1(ReverseLamp)  "<VOUTP_ReverseLamp_flg>"
  [BOUTP_outputs] -> bus_selector59/1
  Ground81/1 -> RoomLampH/1(RoomLampH)
  Ground82/1 -> RoomLampL/1(RoomLampL)
  Ground83/1 -> RrChargingDoorCtrl/1(RrChargingDoorCtrl)
  Ground84/1 -> RrDefog/1(RrDefog)
  bus_selector60/1 -> RrFogLamp/1(RrFogLamp)  "<VOUTP_RrFogLamp_flg>"
  [BOUTP_outputs] -> bus_selector60/1
  Ground85/1 -> RrWiper/1(RrWiper)
  bus_selector61/1 -> ShiftGearPosn/1(ShiftGearPosn)  "<VOUTP_ShiftGearPosn_enum>"
  [BOUTP_outputs] -> bus_selector61/1
  Ground86/1 -> TailgateHDSW/1(TailgateHDSW)
  Ground87/1 -> TailgateRemote/1(TailgateRemote)
  Ground88/1 -> TailgateSW/1(TailgateSW)
  Ground89/1 -> TimeSNDKCFbk/1(TimeSNDKCFbk)
  Ground90/1 -> TrunkRel/1(TrunkRel)
  bus_selector62/1 -> WasherCtrl/1(WasherCtrl)  "<VOUTP_WasherCtrl_enum>"
  [BOUTP_outputs] -> bus_selector62/1
  Ground91/1 -> WiperFixMode/1(WiperFixMode)

== system halout/HAL_OUT/CAN4/FD4_CE100_0_Tx ==
  TxReq : Inport
  BSCP_outputs : Inport  Port=2  OutDataTypeStr=Bus: BSCP_outputs
  BOUTP_outputs : Inport  Port=3  OutDataTypeStr=Bus: BOUTP_outputs
  Chart : Stateflow chart  TreatAsAtomicUnit=on
  Constant : Constant  Value=C_TASK_5MS_S
  Constant3 : Constant  Value=CycleTime
  Data Type Conversion : DataTypeConversion  OutDataTypeStr=uint16
  Divide : Product  Inputs=*/
  Gain : Gain  Gain=0.001
  Ground{,1..52} (53 alike) : Ground
  OR : Logic  Operator=OR  Inputs=76  AllPortsSameDT=off  OutDataTypeStr=boolean
  bus_selector : BusSelector  OutputSignals=VOUTP_APSStaSys_enum
  bus_selector1 : BusSelector  OutputSignals=VOUTP_BrakeLamp_flg
  bus_selector10 : BusSelector  OutputSignals=VOUTP_LDRL_flg
  bus_selector11 : BusSelector  OutputSignals=VOUTP_LTurnLP_flg
  bus_selector12 : BusSelector  OutputSignals=VOUTP_LBeam_flg
  bus_selector13 : BusSelector  OutputSignals=VOUTP_MSACtrlSta_enum
  bus_selector14 : BusSelector  OutputSignals=VOUTP_PosLamp_flg
  bus_selector15 : BusSelector  OutputSignals=VOUTP_PowerSta_enum
  bus_selector16 : BusSelector  OutputSignals=VOUTP_RDRL_flg
  bus_selector17 : BusSelector  OutputSignals=VOUTP_RTurnLP_flg
  bus_selector18 : BusSelector  OutputSignals=VOUTP_ReBrakeLPReq_flg
  bus_selector19 : BusSelector  OutputSignals=VOUTP_ReverseLamp_flg
  bus_selector2 : BusSelector  OutputSignals=VOUTP_CCCtrlSta_enum
  bus_selector20 : BusSelector  OutputSignals=VOUTP_RrFogLamp_flg
  bus_selector21 : BusSelector  OutputSignals=VOUTP_ShiftGearPosn_enum
  bus_selector22 : BusSelector  OutputSignals=VOUTP_WasherCtrl_enum
  bus_selector3 : BusSelector  OutputSignals=VOUTP_DKCAuthSta_enum
  bus_selector4 : BusSelector  OutputSignals=VOUTP_DrSeatSta_enum
  bus_selector5 : BusSelector  OutputSignals=VOUTP_FrWiperH_flg
  bus_selector6 : BusSelector  OutputSignals=VOUTP_FrWiperL_flg
  bus_selector7 : BusSelector  OutputSignals=VOUTP_HBeam_flg
  bus_selector8 : BusSelector  OutputSignals=VOUTP_HazardSW_flg
  bus_selector9 : BusSelector  OutputSignals=VOUTP_HornCtrl_flg
  detect_change{,1..22} (23 alike) : simulink/Logic and Bit Operations/Detect Change  vinit=0  OutDataTypeStr=boolean
  TriggerDataUpdate : Outport
  TriggerCallCDD : Outport  Port=2
  wires:
  Data Type Conversion/1 -> Chart/3(CycleCnt)
  TxReq/1 -> Chart/1(TxReq)
  [EventReq_flg] -> Chart/2(EventReq)
  Constant/1 -> Divide/2
  Divide/1 -> Data Type Conversion/1
  Gain/1 -> Divide/1
  Constant3/1 -> Gain/1
  BSCP_outputs/1 -> [BSCP_outputs]
  BOUTP_outputs/1 -> [BOUTP_outputs]
  OR/1 -> [EventReq_flg]
  detect_change/1 -> OR/1
  bus_selector/1 -> detect_change/1  "<VOUTP_APSStaSys_enum>"
  [BOUTP_outputs] -> bus_selector/1
  Ground/1 -> OR/2
  Ground1/1 -> OR/3
  Ground2/1 -> OR/4
  Ground3/1 -> OR/5
  detect_change1/1 -> OR/6
  bus_selector1/1 -> detect_change1/1  "<VOUTP_BrakeLamp_flg>"
  [BOUTP_outputs] -> bus_selector1/1
  detect_change2/1 -> OR/7
  bus_selector2/1 -> detect_change2/1  "<VOUTP_CCCtrlSta_enum>"
  [BOUTP_outputs] -> bus_selector2/1
  Ground4/1 -> OR/8
  Ground5/1 -> OR/9
  Ground6/1 -> OR/10
  Ground7/1 -> OR/11
  Ground8/1 -> OR/12
  Ground9/1 -> OR/13
  Ground10/1 -> OR/14
  Ground11/1 -> OR/15
  Ground12/1 -> OR/16
  Ground13/1 -> OR/17
  detect_change3/1 -> OR/18
  bus_selector3/1 -> detect_change3/1  "<VOUTP_DKCAuthSta_enum>"
  [BOUTP_outputs] -> bus_selector3/1
  Ground14/1 -> OR/19
  Ground15/1 -> OR/20
  Ground16/1 -> OR/21
  Ground17/1 -> OR/22
  Ground18/1 -> OR/23
  detect_change4/1 -> OR/24
  bus_selector4/1 -> detect_change4/1  "<VOUTP_DrSeatSta_enum>"
  [BOUTP_outputs] -> bus_selector4/1
  Ground19/1 -> OR/25
  Ground20/1 -> OR/26
  Ground21/1 -> OR/27
  Ground22/1 -> OR/28
  Ground23/1 -> OR/29
  Ground24/1 -> OR/30
  Ground25/1 -> OR/31
  Ground26/1 -> OR/32
  Ground27/1 -> OR/33
  detect_change5/1 -> OR/34
  bus_selector5/1 -> detect_change5/1  "<VOUTP_FrWiperH_flg>"
  [BOUTP_outputs] -> bus_selector5/1
  detect_change6/1 -> OR/35
  bus_selector6/1 -> detect_change6/1  "<VOUTP_FrWiperL_flg>"
  [BOUTP_outputs] -> bus_selector6/1
  Ground28/1 -> OR/36
  detect_change7/1 -> OR/37
  bus_selector7/1 -> detect_change7/1  "<VOUTP_HBeam_flg>"
  [BOUTP_outputs] -> bus_selector7/1
  Ground29/1 -> OR/38
  detect_change8/1 -> OR/39
  bus_selector8/1 -> detect_change8/1  "<VOUTP_HazardSW_flg>"
  [BOUTP_outputs] -> bus_selector8/1
  Ground30/1 -> OR/40
  detect_change9/1 -> OR/41
  bus_selector9/1 -> detect_change9/1  "<VOUTP_HornCtrl_flg>"
  [BOUTP_outputs] -> bus_selector9/1
  Ground31/1 -> OR/42
  detect_change10/1 -> OR/43
  bus_selector10/1 -> detect_change10/1  "<VOUTP_LDRL_flg>"
  [BOUTP_outputs] -> bus_selector10/1
  detect_change11/1 -> OR/44
  bus_selector11/1 -> detect_change11/1  "<VOUTP_LTurnLP_flg>"
  [BOUTP_outputs] -> bus_selector11/1
  Ground32/1 -> OR/45
  detect_change12/1 -> OR/46
  bus_selector12/1 -> detect_change12/1  "<VOUTP_LBeam_flg>"
  [BOUTP_outputs] -> bus_selector12/1
  Ground33/1 -> OR/47
  Ground34/1 -> OR/48
  detect_change13/1 -> OR/49
  bus_selector13/1 -> detect_change13/1  "<VOUTP_MSACtrlSta_enum>"
  [BOUTP_outputs] -> bus_selector13/1
  Ground35/1 -> OR/50
  Ground36/1 -> OR/51
  detect_change14/1 -> OR/52
  bus_selector14/1 -> detect_change14/1  "<VOUTP_PosLamp_flg>"
  [BOUTP_outputs] -> bus_selector14/1
  Ground37/1 -> OR/53
  detect_change15/1 -> OR/54
  bus_selector15/1 -> detect_change15/1  "<VOUTP_PowerSta_enum>"
  [BOUTP_outputs] -> bus_selector15/1
  Ground38/1 -> OR/55
  Ground39/1 -> OR/56
  detect_change16/1 -> OR/57
  bus_selector16/1 -> detect_change16/1  "<VOUTP_RDRL_flg>"
  [BOUTP_outputs] -> bus_selector16/1
  Ground40/1 -> OR/58
  Ground41/1 -> OR/59
  detect_change17/1 -> OR/60
  bus_selector17/1 -> detect_change17/1  "<VOUTP_RTurnLP_flg>"
  [BOUTP_outputs] -> bus_selector17/1
  detect_change18/1 -> OR/61
  bus_selector18/1 -> detect_change18/1  "<VOUTP_ReBrakeLPReq_flg>"
  [BOUTP_outputs] -> bus_selector18/1
  detect_change19/1 -> OR/62
  bus_selector19/1 -> detect_change19/1  "<VOUTP_ReverseLamp_flg>"
  [BOUTP_outputs] -> bus_selector19/1
  Ground42/1 -> OR/63
  Ground43/1 -> OR/64
  Ground44/1 -> OR/65
  Ground45/1 -> OR/66
  detect_change20/1 -> OR/67
  bus_selector20/1 -> detect_change20/1  "<VOUTP_RrFogLamp_flg>"
  [BOUTP_outputs] -> bus_selector20/1
  Ground46/1 -> OR/68
  detect_change21/1 -> OR/69
  bus_selector21/1 -> detect_change21/1  "<VOUTP_ShiftGearPosn_enum>"
  [BOUTP_outputs] -> bus_selector21/1
  Ground47/1 -> OR/70
  Ground48/1 -> OR/71
  Ground49/1 -> OR/72
  Ground50/1 -> OR/73
  Ground51/1 -> OR/74
  detect_change22/1 -> OR/75
  bus_selector22/1 -> detect_change22/1  "<VOUTP_WasherCtrl_enum>"
  [BOUTP_outputs] -> bus_selector22/1
  Ground52/1 -> OR/76
  Chart/2(TriggerCallCDD()) -> TriggerCallCDD/1
  Chart/1(TriggerDataUpdate()) -> TriggerDataUpdate/1
